simulink model "laplace_sin"  (R2024b)
settings: Solver=VariableStepAuto  StartTime=0.0  StopTime=10.0  RelTol=1e-3
settings Model: Creator=omari  LastModifiedBy=omari

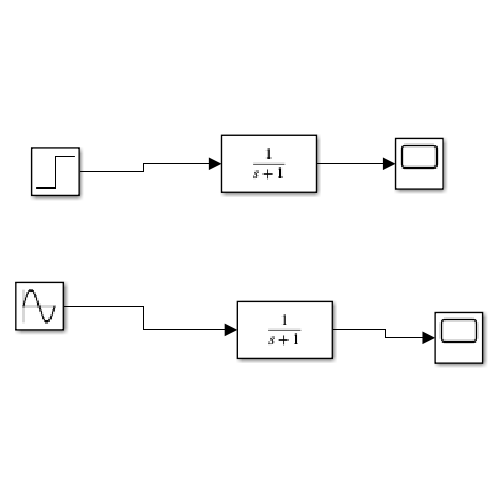
[thumbnail: Simulink's stored preview of the top-level diagram]
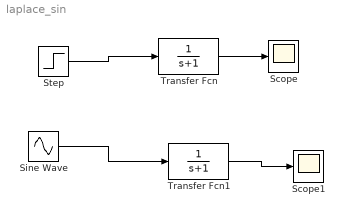
== system laplace_sin ==
  Scope : Scope
  Scope1 : Scope
  Sine Wave : Sin  Amplitude=5  SampleTime=0
  Step : Step  SampleTime=0
  Transfer Fcn : TransferFcn  Denominator=[1 1]
  Transfer Fcn1 : TransferFcn  Denominator=[1 1]
  wires:
  Step/1 -> Transfer Fcn/1
  Transfer Fcn/1 -> Scope/1
  Sine Wave/1 -> Transfer Fcn1/1
  Transfer Fcn1/1 -> Scope1/1
